simulink model "OMAP"  (R2018b)
settings: Solver=FixedStepDiscrete  StartTime=0.0  StopTime=10.0  FixedStep=0.01  RelTol=1e-3
values from neighbouring files (symbols this model uses):
  Clb_ICADirect_LaneDisp_StateFive = Simulink.Parameter    [omap_ver_442.m]
  Clb_ICADirect_LaneDisp_StateFour = Simulink.Parameter    [omap_ver_442.m]
  Clb_ICADirect_LaneDisp_StateOne = Simulink.Parameter    [omap_ver_442.m]
  Clb_ICADirect_LaneDisp_StateThree = Simulink.Parameter    [omap_ver_442.m]
  Clb_ICADirect_LaneDisp_StateTwo = Simulink.Parameter    [omap_ver_442.m]
  Clb_ICADirect_LaneDisp_StateZero = Simulink.Parameter    [omap_ver_442.m]
  Clb_ICADirect_LaneDispSW = Simulink.Parameter    [omap_ver_442.m]
  Clb_ICADirect_TrnLghtsCom_Switch = Simulink.Parameter    [omap_ver_442.m]
  Clb_ICADirect_TrnLghtsCom_Value = Simulink.Parameter    [omap_ver_442.m]
  Clb_ICADirect_TrnLghtsCrtl_Inhb = Simulink.Parameter    [omap_ver_442.m]
  OMAP_ACCAEB_EMSESC_Decel = Simulink.Parameter    [omap_ver_442.m]
  OMAP_ACCFCW_IC_Decel = Simulink.Parameter    [omap_ver_442.m]
  OMAP_clb_ACC_RVVReqType = Simulink.Parameter    [omap_ver_442.m]
  OMAP_clb_ACC_RVVReqType_Switch = Simulink.Parameter    [omap_ver_442.m]
  OMAP_clb_ACCHeadwayDisplay = Simulink.Parameter    [omap_ver_442.m]
  OMAP_clb_ACCHeadwayDisplay_Switch = Simulink.Parameter    [omap_ver_442.m]
  OMAP_clb_ACCHeadwayIcon = Simulink.Parameter    [omap_ver_442.m]
  OMAP_clb_ACCHeadwayIcon_Switch = Simulink.Parameter    [omap_ver_442.m]
  OMAP_clb_ACCMessagePrompt = Simulink.Parameter    [omap_ver_442.m]
  OMAP_clb_ACCMessagePrompt_Switch = Simulink.Parameter    [omap_ver_442.m]
  OMAP_clb_ACCRequestEPB = Simulink.Parameter    [omap_ver_442.m]
  OMAP_clb_ACCRequestEPB_Switch = Simulink.Parameter    [omap_ver_442.m]
  OMAP_clb_ACCSetSpeed = Simulink.Parameter    [omap_ver_442.m]
  OMAP_clb_ACCSetSpeed_Switch = Simulink.Parameter    [omap_ver_442.m]
  OMAP_clb_ACCSetSpeedDis = Simulink.Parameter    [omap_ver_442.m]
  OMAP_clb_ACCSetSpeedDis_Switch = Simulink.Parameter    [omap_ver_442.m]
  OMAP_clb_ACCState = Simulink.Parameter    [omap_ver_442.m]
  OMAP_clb_ACCState_Switch = Simulink.Parameter    [omap_ver_442.m]
  OMAP_clb_ACCStatusIconDis = Simulink.Parameter    [omap_ver_442.m]
  OMAP_clb_ACCStatusIconDis_Switch = Simulink.Parameter    [omap_ver_442.m]
  OMAP_clb_ACCTorqueReq = Simulink.Parameter    [omap_ver_442.m]
  OMAP_clb_ACCTorqueReq_Switch = Simulink.Parameter    [omap_ver_442.m]
  OMAP_clb_ADAS_State = Simulink.Parameter    [omap_ver_442.m]
  OMAP_clb_ADAS_State_Switch = Simulink.Parameter    [omap_ver_442.m]
  OMAP_clb_AEBAlertReq = Simulink.Parameter    [omap_ver_442.m]
  OMAP_clb_AEBAlertReq_Switch = Simulink.Parameter    [omap_ver_442.m]
  OMAP_clb_AEBBrakingProg = Simulink.Parameter    [omap_ver_442.m]
  OMAP_clb_AEBBrakingProg_Switch = Simulink.Parameter    [omap_ver_442.m]
  OMAP_clb_AEBFaultStatus = Simulink.Parameter    [omap_ver_442.m]
  OMAP_clb_AEBFaultStatus_Switch = Simulink.Parameter    [omap_ver_442.m]
  OMAP_clb_AEBMassageDisp = Simulink.Parameter    [omap_ver_442.m]
  OMAP_clb_AEBMassageDisp_Switch = Simulink.Parameter    [omap_ver_442.m]
  OMAP_clb_AEBState = Simulink.Parameter    [omap_ver_442.m]
  OMAP_clb_AEBState_Switch = Simulink.Parameter    [omap_ver_442.m]
  OMAP_clb_AEBSwitchStatus = Simulink.Parameter    [omap_ver_442.m]
  OMAP_clb_AEBSwitchStatus_Switch = Simulink.Parameter    [omap_ver_442.m]
  OMAP_clb_BrakeRequest = Simulink.Parameter    [omap_ver_442.m]
  OMAP_clb_BrakeRequest_Switch = Simulink.Parameter    [omap_ver_442.m]
  OMAP_clb_DecelerationSet = Simulink.Parameter    [omap_ver_442.m]
  OMAP_clb_DecelerationSet_Switch = Simulink.Parameter    [omap_ver_442.m]
  OMAP_clb_DecelerationType = Simulink.Parameter    [omap_ver_442.m]
  OMAP_clb_DecelerationType_Switch = Simulink.Parameter    [omap_ver_442.m]
  OMAP_clb_DeclControlReq = Simulink.Parameter    [omap_ver_442.m]
  OMAP_clb_DeclControlReq_Switch = Simulink.Parameter    [omap_ver_442.m]
  OMAP_clb_DownorUpGearMinTime = Simulink.Parameter    [omap_ver_442.m]
  OMAP_clb_DownorUpGearMinTime_Switch = Simulink.Parameter    [omap_ver_442.m]
  OMAP_clb_ELKPopupMessage = Simulink.Parameter    [omap_ver_442.m]
  OMAP_clb_ELKPopupMessage_Switch = Simulink.Parameter    [omap_ver_442.m]
  OMAP_clb_ELKSts = Simulink.Parameter    [omap_ver_442.m]
  OMAP_clb_ELKSts_Switch = Simulink.Parameter    [omap_ver_442.m]
  OMAP_clb_ESAFaultSt = Simulink.Parameter    [omap_ver_442.m]
  OMAP_clb_ESAFaultSt_Switch = Simulink.Parameter    [omap_ver_442.m]
  OMAP_clb_ESARequest = Simulink.Parameter    [omap_ver_442.m]
  OMAP_clb_ESARequest_Switch = Simulink.Parameter    [omap_ver_442.m]
  OMAP_clb_ESAState = Simulink.Parameter    [omap_ver_442.m]
  OMAP_clb_ESAState_Switch = Simulink.Parameter    [omap_ver_442.m]
  OMAP_clb_ESATorqueReq = Simulink.Parameter    [omap_ver_442.m]
  OMAP_clb_ESATorqueReq_Switch = Simulink.Parameter    [omap_ver_442.m]
  OMAP_clb_ESCDriveOff = Simulink.Parameter    [omap_ver_442.m]
  OMAP_clb_ESCDriveOff_Switch = Simulink.Parameter    [omap_ver_442.m]
  OMAP_clb_ESCHoldReq = Simulink.Parameter    [omap_ver_442.m]
  OMAP_clb_ESCHoldReq_Switch = Simulink.Parameter    [omap_ver_442.m]
  OMAP_clb_Handsoffwarning = Simulink.Parameter    [omap_ver_442.m]
  OMAP_clb_Handsoffwarning_Switch = Simulink.Parameter    [omap_ver_442.m]
  OMAP_clb_HapticAlarmReq = Simulink.Parameter    [omap_ver_442.m]
  OMAP_clb_HapticAlarmReq_Switch = Simulink.Parameter    [omap_ver_442.m]
  OMAP_clb_HMIPopupMassage = Simulink.Parameter    [omap_ver_442.m]
  OMAP_clb_HMIPopupMassage_Switch = Simulink.Parameter    [omap_ver_442.m]
  OMAP_clb_HWAActionSts = Simulink.Parameter    [omap_ver_442.m]
  OMAP_clb_HWAActionSts_Switch = Simulink.Parameter    [omap_ver_442.m]
  OMAP_clb_HWAMode = Simulink.Parameter    [omap_ver_442.m]
  OMAP_clb_HWAMode_Switch = Simulink.Parameter    [omap_ver_442.m]
  OMAP_clb_HWATurnOnIdctr = Simulink.Parameter    [omap_ver_442.m]
  OMAP_clb_HWATurnOnIdctr_Switch = Simulink.Parameter    [omap_ver_442.m]
  OMAP_clb_ICAMassageDisp = Simulink.Parameter    [omap_ver_442.m]
  OMAP_clb_ICAMassageDisp_Switch = Simulink.Parameter    [omap_ver_442.m]
  OMAP_clb_ICAStatusIcon = Simulink.Parameter    [omap_ver_442.m]
  OMAP_clb_ICAStatusIcon_Switch = Simulink.Parameter    [omap_ver_442.m]
  OMAP_clb_ISLCDriverRemind = Simulink.Parameter    [omap_ver_442.m]
  OMAP_clb_ISLCDriverRemind_Switch = Simulink.Parameter    [omap_ver_442.m]
  OMAP_clb_ISLCState = Simulink.Parameter    [omap_ver_442.m]
  OMAP_clb_ISLCState_Switch = Simulink.Parameter    [omap_ver_442.m]
  OMAP_clb_JAFaultSt = Simulink.Parameter    [omap_ver_442.m]
  OMAP_clb_JAFaultSt_Switch = Simulink.Parameter    [omap_ver_442.m]
  OMAP_clb_LCAPopupMessage = Simulink.Parameter    [omap_ver_442.m]
  OMAP_clb_LCAPopupMessage_Switch = Simulink.Parameter    [omap_ver_442.m]
  OMAP_clb_LCAStatusDisplay = Simulink.Parameter    [omap_ver_442.m]
  OMAP_clb_LCAStatusDisplay_Switch = Simulink.Parameter    [omap_ver_442.m]
  OMAP_clb_LDWStatusDisplay = Simulink.Parameter    [omap_ver_442.m]
  OMAP_clb_LDWStatusDisplay_Switch = Simulink.Parameter    [omap_ver_442.m]
  OMAP_clb_LDWWarningSt = Simulink.Parameter    [omap_ver_442.m]
  OMAP_clb_LDWWarningSt_Switch = Simulink.Parameter    [omap_ver_442.m]
  OMAP_clb_LightControlValid = Simulink.Parameter    [omap_ver_442.m]
  OMAP_clb_LightControlValid_Switch = Simulink.Parameter    [omap_ver_442.m]
  OMAP_clb_LKAActivation = Simulink.Parameter    [omap_ver_442.m]
  OMAP_clb_LKAActivation_Switch = Simulink.Parameter    [omap_ver_442.m]
  OMAP_clb_LKAAngleReq = Simulink.Parameter    [omap_ver_442.m]
  OMAP_clb_LKAAngleReq_Switch = Simulink.Parameter    [omap_ver_442.m]
  OMAP_clb_LKAMode = Simulink.Parameter    [omap_ver_442.m]
  OMAP_clb_LKAMode_Switch = Simulink.Parameter    [omap_ver_442.m]
  OMAP_clb_LKAorELK_CoolTime = Simulink.Parameter    [omap_ver_442.m]
  OMAP_clb_LKAState = Simulink.Parameter    [omap_ver_442.m]
  OMAP_clb_LKAState_Switch = Simulink.Parameter    [omap_ver_442.m]
  OMAP_clb_LKAStatusDisplay = Simulink.Parameter    [omap_ver_442.m]
  OMAP_clb_LKAStatusDisplay_Switch = Simulink.Parameter    [omap_ver_442.m]
  OMAP_clb_LKASwitchState = Simulink.Parameter    [omap_ver_442.m]
  OMAP_clb_LKASwitchState_Switch = Simulink.Parameter    [omap_ver_442.m]
  OMAP_clb_LKATorqFactReq = Simulink.Parameter    [omap_ver_442.m]
  OMAP_clb_LKATorqFactReq_Switch = Simulink.Parameter    [omap_ver_442.m]
  OMAP_clb_PrefillRequest = Simulink.Parameter    [omap_ver_442.m]
  ... (+36 more)
libraries: simulink x184, canmsglib x2
(part 14 of 14)

== system OMAP/Runnable_OMAP_10ms_sys/OMAP_Module/ICA_Direct_G59/ICA_Define/Subsystem1/Dspl/DsplPrcs/Txt/TxtFromACC/RdrBlkInhib ==
  RdrBlkInhib_stTHState : Inport
  RdrBlkInhib_stLstTHState : Inport  Port=2
  RdrBlkInhib_stACCTxtDspl : Inport  Port=3
  Constant1 : Constant  OutDataTypeStr=uint16
  Constant2 : Constant  Value=0  OutDataTypeStr=uint16
  If : If  NumInputs=3  IfExpression=u1 == 5 & u2 == 0 & u3 == 2  ElseIfExpressions=u1 ~= 5 | u3 ~= 2
  Inhibit : Subsystem  TreatAsAtomicUnit=on
  Merge : Merge  Inputs=3
  Unit Delay1 : UnitDelay  SampleTime=-1
  hold_last : Subsystem  TreatAsAtomicUnit=on
  not_Inhibit : Subsystem  TreatAsAtomicUnit=on
  RdrBlkInhib_stRdrBlkInhibFlg : Outport
  wires:
  RdrBlkInhib_stTHState/1 -> If/1
  Merge/1 -> Unit Delay1/1, RdrBlkInhib_stRdrBlkInhibFlg/1
  Inhibit/1(Out1) -> Merge/1
  RdrBlkInhib_stLstTHState/1 -> If/2
  RdrBlkInhib_stACCTxtDspl/1 -> If/3
  Constant1/1 -> Inhibit/1(In1)
  If/1 -> Inhibit/Action
  Constant2/1 -> not_Inhibit/1(In1)
  If/2 -> not_Inhibit/Action
  Unit Delay1/1 -> hold_last/1(In1)
  If/3 -> hold_last/Action
  not_Inhibit/1(Out1) -> Merge/2
  hold_last/1(Out1) -> Merge/3

== system OMAP/Runnable_OMAP_10ms_sys/OMAP_Module/ICA_Direct_G59/ICA_Define/Subsystem1/Dspl/DsplPrcs/Txt/TxtFromACC/Start ==
  In1 : Inport
  Action Port : ActionPort  ActionType=then
  Out1 : Outport
  wires:
  In1/1 -> Out1/1

== system OMAP/Runnable_OMAP_10ms_sys/OMAP_Module/ICA_Direct_G59/ICA_Define/Subsystem1/Dspl/DsplPrcs/Txt/TxtFromACC/Start1 ==
  In1 : Inport
  Action Port : ActionPort  ActionType=then
  Out1 : Outport
  wires:
  In1/1 -> Out1/1

== system OMAP/Runnable_OMAP_10ms_sys/OMAP_Module/ICA_Direct_G59/ICA_Define/Subsystem1/Dspl/DsplPrcs/Txt/TxtFromACC/Start2 ==
  In1 : Inport
  Action Port : ActionPort  ActionType=then
  Out1 : Outport
  wires:
  In1/1 -> Out1/1

== system OMAP/Runnable_OMAP_10ms_sys/OMAP_Module/ICA_Direct_G59/ICA_Define/Subsystem1/Dspl/DsplPrcs/Txt/TxtFromACC/Start3 ==
  In1 : Inport
  Action Port : ActionPort  ActionType=then
  Out1 : Outport
  wires:
  In1/1 -> Out1/1

== system OMAP/Runnable_OMAP_10ms_sys/OMAP_Module/ICA_Direct_G59/ICA_Define/Subsystem1/Dspl/DsplPrcs/Txt/TxtFromACC/Start4 ==
  In1 : Inport
  Action Port : ActionPort  ActionType=then
  Out1 : Outport
  wires:
  In1/1 -> Out1/1

== system OMAP/Runnable_OMAP_10ms_sys/OMAP_Module/ICA_Direct_G59/ICA_Define/Subsystem1/Dspl/DsplPrcs/Txt/TxtFromACC/Start5 ==
  In1 : Inport
  Action Port : ActionPort  ActionType=then
  Out1 : Outport
  wires:
  In1/1 -> Out1/1

== system OMAP/Runnable_OMAP_10ms_sys/OMAP_Module/ICA_Direct_G59/ICA_Define/Subsystem1/Dspl/DsplPrcs/Txt/TxtFromACC/Start6 ==
  In1 : Inport
  Action Port : ActionPort  ActionType=then
  Out1 : Outport
  wires:
  In1/1 -> Out1/1

== system OMAP/Runnable_OMAP_10ms_sys/OMAP_Module/ICA_Direct_G59/ICA_Define/Subsystem1/Dspl/DsplPrcs/Txt/TxtFromACC/Start7 ==
  In1 : Inport
  Action Port : ActionPort  ActionType=then
  Out1 : Outport
  wires:
  In1/1 -> Out1/1

== system OMAP/Runnable_OMAP_10ms_sys/OMAP_Module/ICA_Direct_G59/ICA_Define/Subsystem1/Dspl/DsplPrcs/Txt/TxtFromACC/Start8 ==
  In1 : Inport
  Action Port : ActionPort  ActionType=then
  Out1 : Outport
  wires:
  In1/1 -> Out1/1

== system OMAP/Runnable_OMAP_10ms_sys/OMAP_Module/ICA_Direct_G59/ICA_Define/Subsystem1/Dspl/DsplPrcs/Txt/TxtFromACC/Start9 ==
  In1 : Inport
  Action Port : ActionPort  ActionType=then
  Out1 : Outport
  wires:
  In1/1 -> Out1/1

== system OMAP/Runnable_OMAP_10ms_sys/OMAP_Module/ICA_Direct_G59/ICA_Define/Subsystem1/Dspl/DsplPrcs/Txt/TxtFromACC/Stop ==
  In1 : Inport
  Action Port : ActionPort  ActionType=else
  Out1 : Outport
  wires:
  In1/1 -> Out1/1

== system OMAP/Runnable_OMAP_10ms_sys/OMAP_Module/ICA_Direct_G59/ICA_Define/Subsystem1/Dspl/DsplPrcs/Txt/TxtFromACC/Stop1 ==
  In1 : Inport
  Action Port : ActionPort  ActionType=else
  Out1 : Outport
  wires:
  In1/1 -> Out1/1

== system OMAP/Runnable_OMAP_10ms_sys/OMAP_Module/ICA_Direct_G59/ICA_Define/Subsystem1/Dspl/DsplPrcs/Txt/TxtFromACC/Stop2 ==
  In1 : Inport
  Action Port : ActionPort  ActionType=else
  Out1 : Outport
  wires:
  In1/1 -> Out1/1

== system OMAP/Runnable_OMAP_10ms_sys/OMAP_Module/ICA_Direct_G59/ICA_Define/Subsystem1/Dspl/DsplPrcs/Txt/TxtFromACC/Stop3 ==
  In1 : Inport
  Action Port : ActionPort  ActionType=else
  Out1 : Outport
  wires:
  In1/1 -> Out1/1

== system OMAP/Runnable_OMAP_10ms_sys/OMAP_Module/ICA_Direct_G59/ICA_Define/Subsystem1/Dspl/DsplPrcs/Txt/TxtFromACC/Stop4 ==
  In1 : Inport
  Action Port : ActionPort  ActionType=elseif
  Out1 : Outport
  wires:
  In1/1 -> Out1/1

== system OMAP/Runnable_OMAP_10ms_sys/OMAP_Module/ICA_Direct_G59/ICA_Define/Subsystem1/Dspl/DsplPrcs/Txt/TxtFromACC/Stop5 ==
  In1 : Inport
  Action Port : ActionPort  ActionType=else
  Out1 : Outport
  wires:
  In1/1 -> Out1/1

== system OMAP/Runnable_OMAP_10ms_sys/OMAP_Module/ICA_Direct_G59/ICA_Define/Subsystem1/Dspl/DsplPrcs/Txt/TxtFromACC/Stop6 ==
  In1 : Inport
  Action Port : ActionPort  ActionType=else
  Out1 : Outport
  wires:
  In1/1 -> Out1/1

== system OMAP/Runnable_OMAP_10ms_sys/OMAP_Module/ICA_Direct_G59/ICA_Define/Subsystem1/Dspl/DsplPrcs/Txt/TxtFromACC/Stop7 ==
  In1 : Inport
  Action Port : ActionPort  ActionType=else
  Out1 : Outport
  wires:
  In1/1 -> Out1/1

== system OMAP/Runnable_OMAP_10ms_sys/OMAP_Module/ICA_Direct_G59/ICA_Define/Subsystem1/Dspl/DsplPrcs/Txt/TxtFromACC/Stop8 ==
  In1 : Inport
  Action Port : ActionPort  ActionType=else
  Out1 : Outport
  wires:
  In1/1 -> Out1/1

== system OMAP/Runnable_OMAP_10ms_sys/OMAP_Module/ICA_Direct_G59/ICA_Define/Subsystem1/Dspl/DsplPrcs/Txt/TxtFromACC/Stop9 ==
  In1 : Inport
  Action Port : ActionPort  ActionType=else
  Out1 : Outport
  wires:
  In1/1 -> Out1/1

== system OMAP/Runnable_OMAP_10ms_sys/OMAP_Module/ICA_Direct_G59/ICA_Define/Subsystem1/Dspl/DsplPrcs/Txt/TxtInactv/Hold ==
  In1 : Inport
  Action Port : ActionPort  ActionType=else
  Out1 : Outport
  wires:
  In1/1 -> Out1/1

== system OMAP/Runnable_OMAP_10ms_sys/OMAP_Module/ICA_Direct_G59/ICA_Define/Subsystem1/Dspl/DsplPrcs/Txt/TxtInactv/Start ==
  In1 : Inport
  Action Port : ActionPort  ActionType=elseif
  Out1 : Outport
  wires:
  In1/1 -> Out1/1

== system OMAP/Runnable_OMAP_10ms_sys/OMAP_Module/ICA_Direct_G59/ICA_Define/Subsystem1/Dspl/DsplPrcs/Txt/TxtInactv/Stop ==
  In1 : Inport
  Action Port : ActionPort  ActionType=then
  Out1 : Outport
  wires:
  In1/1 -> Out1/1

== system OMAP/Runnable_OMAP_10ms_sys/OMAP_Module/ICA_Direct_G59/ICA_Define/Subsystem1/Dspl/DsplPrcs/Txt/TxtOff/Hold ==
  In1 : Inport
  Action Port : ActionPort  ActionType=else
  Out1 : Outport
  wires:
  In1/1 -> Out1/1

== system OMAP/Runnable_OMAP_10ms_sys/OMAP_Module/ICA_Direct_G59/ICA_Define/Subsystem1/Dspl/DsplPrcs/Txt/TxtOff/Start ==
  In1 : Inport
  Action Port : ActionPort  ActionType=then
  Out1 : Outport
  wires:
  In1/1 -> Out1/1

== system OMAP/Runnable_OMAP_10ms_sys/OMAP_Module/ICA_Direct_G59/ICA_Define/Subsystem1/Dspl/DsplPrcs/Txt/TxtOff/Stop ==
  In1 : Inport
  Action Port : ActionPort  ActionType=elseif
  Out1 : Outport
  wires:
  In1/1 -> Out1/1

== system OMAP/Runnable_OMAP_10ms_sys/OMAP_Module/ICA_Direct_G59/ICA_Define/Subsystem1/Dspl/DsplPrcs/Txt/TxtOffToFault/Hold ==
  In1 : Inport
  Action Port : ActionPort  ActionType=else
  Out1 : Outport
  wires:
  In1/1 -> Out1/1

== system OMAP/Runnable_OMAP_10ms_sys/OMAP_Module/ICA_Direct_G59/ICA_Define/Subsystem1/Dspl/DsplPrcs/Txt/TxtOffToFault/Start ==
  In1 : Inport
  Action Port : ActionPort  ActionType=then
  Out1 : Outport
  wires:
  In1/1 -> Out1/1

== system OMAP/Runnable_OMAP_10ms_sys/OMAP_Module/ICA_Direct_G59/ICA_Define/Subsystem1/Dspl/DsplPrcs/Txt/TxtOffToFault/Stop ==
  In1 : Inport
  Action Port : ActionPort  ActionType=elseif
  Out1 : Outport
  wires:
  In1/1 -> Out1/1

== system OMAP/Runnable_OMAP_10ms_sys/OMAP_Module/ICA_Direct_G59/ICA_Define/Subsystem1/Dspl/DsplPrcs/Txt/TxtOn/Hold ==
  In1 : Inport
  Action Port : ActionPort  ActionType=else
  Out1 : Outport
  wires:
  In1/1 -> Out1/1

== system OMAP/Runnable_OMAP_10ms_sys/OMAP_Module/ICA_Direct_G59/ICA_Define/Subsystem1/Dspl/DsplPrcs/Txt/TxtOn/Start ==
  In1 : Inport
  Action Port : ActionPort  ActionType=then
  Out1 : Outport
  wires:
  In1/1 -> Out1/1

== system OMAP/Runnable_OMAP_10ms_sys/OMAP_Module/ICA_Direct_G59/ICA_Define/Subsystem1/Dspl/DsplPrcs/Txt/TxtOn/Stop ==
  In1 : Inport
  Action Port : ActionPort  ActionType=elseif
  Out1 : Outport
  wires:
  In1/1 -> Out1/1

== system OMAP/Runnable_OMAP_10ms_sys/OMAP_Module/ICA_Direct_G59/ICA_Define/Subsystem1/Dspl/DsplPrcs/Txt/TxtOnToFault/Hold ==
  In1 : Inport
  Action Port : ActionPort  ActionType=else
  Out1 : Outport
  wires:
  In1/1 -> Out1/1

== system OMAP/Runnable_OMAP_10ms_sys/OMAP_Module/ICA_Direct_G59/ICA_Define/Subsystem1/Dspl/DsplPrcs/Txt/TxtOnToFault/Start ==
  In1 : Inport
  Action Port : ActionPort  ActionType=then
  Out1 : Outport
  wires:
  In1/1 -> Out1/1

== system OMAP/Runnable_OMAP_10ms_sys/OMAP_Module/ICA_Direct_G59/ICA_Define/Subsystem1/Dspl/DsplPrcs/Txt/TxtOnToFault/Stop ==
  In1 : Inport
  Action Port : ActionPort  ActionType=elseif
  Out1 : Outport
  wires:
  In1/1 -> Out1/1

== system OMAP/Runnable_OMAP_10ms_sys/OMAP_Module/ICA_Direct_G59/ICA_Define/Subsystem1/Dspl/DsplPrcs/Txt/Txt_Tlimit/Hold ==
  In1 : Inport
  Action Port : ActionPort  ActionType=else
  Out1 : Outport
  wires:
  In1/1 -> Out1/1

== system OMAP/Runnable_OMAP_10ms_sys/OMAP_Module/ICA_Direct_G59/ICA_Define/Subsystem1/Dspl/DsplPrcs/Txt/Txt_Tlimit/Start ==
  In1 : Inport
  Action Port : ActionPort  ActionType=then
  Out1 : Outport
  wires:
  In1/1 -> Out1/1

== system OMAP/Runnable_OMAP_10ms_sys/OMAP_Module/ICA_Direct_G59/ICA_Define/Subsystem1/Dspl/DsplPrcs/Txt/Txt_Tlimit/Stop ==
  In1 : Inport
  Action Port : ActionPort  ActionType=elseif
  Out1 : Outport
  wires:
  In1/1 -> Out1/1

== system OMAP/Runnable_OMAP_10ms_sys/OMAP_Module/ICA_Direct_G59/ICA_Define/Subsystem1/Dspl/DsplPrcs/Txt/Txt_Tlimit1/Hold ==
  In1 : Inport
  Action Port : ActionPort  ActionType=else
  Out1 : Outport
  wires:
  In1/1 -> Out1/1

== system OMAP/Runnable_OMAP_10ms_sys/OMAP_Module/ICA_Direct_G59/ICA_Define/Subsystem1/Dspl/DsplPrcs/Txt/Txt_Tlimit1/Start ==
  In1 : Inport
  Action Port : ActionPort  ActionType=then
  Out1 : Outport
  wires:
  In1/1 -> Out1/1

== system OMAP/Runnable_OMAP_10ms_sys/OMAP_Module/ICA_Direct_G59/ICA_Define/Subsystem1/Dspl/DsplPrcs/Txt/Txt_Tlimit1/Stop ==
  In1 : Inport
  Action Port : ActionPort  ActionType=elseif
  Out1 : Outport
  wires:
  In1/1 -> Out1/1

== system OMAP/Runnable_OMAP_10ms_sys/OMAP_Module/ICA_Direct_G59/ICA_Define/Subsystem1/Dspl/DsplPrcs/Txt/Txt_Tlimit2/Hold ==
  In1 : Inport
  Action Port : ActionPort  ActionType=else
  Out1 : Outport
  wires:
  In1/1 -> Out1/1

== system OMAP/Runnable_OMAP_10ms_sys/OMAP_Module/ICA_Direct_G59/ICA_Define/Subsystem1/Dspl/DsplPrcs/Txt/Txt_Tlimit2/Start ==
  In1 : Inport
  Action Port : ActionPort  ActionType=then
  Out1 : Outport
  wires:
  In1/1 -> Out1/1

== system OMAP/Runnable_OMAP_10ms_sys/OMAP_Module/ICA_Direct_G59/ICA_Define/Subsystem1/Dspl/DsplPrcs/Txt/Txt_Tlimit2/Stop ==
  In1 : Inport
  Action Port : ActionPort  ActionType=elseif
  Out1 : Outport
  wires:
  In1/1 -> Out1/1

== system OMAP/Runnable_OMAP_10ms_sys/OMAP_Module/ICA_Direct_G59/ICA_Define/Subsystem1/Dspl/DsplPrcs/Txt/Txt_Tlimit3/Hold ==
  In1 : Inport
  Action Port : ActionPort  ActionType=else
  Out1 : Outport
  wires:
  In1/1 -> Out1/1

== system OMAP/Runnable_OMAP_10ms_sys/OMAP_Module/ICA_Direct_G59/ICA_Define/Subsystem1/Dspl/DsplPrcs/Txt/Txt_Tlimit3/Start ==
  In1 : Inport
  Action Port : ActionPort  ActionType=then
  Out1 : Outport
  wires:
  In1/1 -> Out1/1

== system OMAP/Runnable_OMAP_10ms_sys/OMAP_Module/ICA_Direct_G59/ICA_Define/Subsystem1/Dspl/DsplPrcs/Txt/Txt_Tlimit3/Stop ==
  In1 : Inport
  Action Port : ActionPort  ActionType=elseif
  Out1 : Outport
  wires:
  In1/1 -> Out1/1

== system OMAP/Runnable_OMAP_10ms_sys/OMAP_Module/ICA_Direct_G59/ICA_Define/Subsystem1/Dspl/DsplPrcs/Txt/Txt_Tlimit4/Hold ==
  In1 : Inport
  Action Port : ActionPort  ActionType=else
  Out1 : Outport
  wires:
  In1/1 -> Out1/1

== system OMAP/Runnable_OMAP_10ms_sys/OMAP_Module/ICA_Direct_G59/ICA_Define/Subsystem1/Dspl/DsplPrcs/Txt/Txt_Tlimit4/Start ==
  In1 : Inport
  Action Port : ActionPort  ActionType=then
  Out1 : Outport
  wires:
  In1/1 -> Out1/1

== system OMAP/Runnable_OMAP_10ms_sys/OMAP_Module/ICA_Direct_G59/ICA_Define/Subsystem1/Dspl/DsplPrcs/Txt/Txt_Tlimit4/Stop ==
  In1 : Inport
  Action Port : ActionPort  ActionType=elseif
  Out1 : Outport
  wires:
  In1/1 -> Out1/1

== system OMAP/Runnable_OMAP_10ms_sys/OMAP_Module/ICA_Direct_G59/ICA_Define/Subsystem1/Dspl/DsplPrcs/Txt/Txt_Tlimit5/Hold ==
  In1 : Inport
  Action Port : ActionPort  ActionType=else
  Out1 : Outport
  wires:
  In1/1 -> Out1/1

== system OMAP/Runnable_OMAP_10ms_sys/OMAP_Module/ICA_Direct_G59/ICA_Define/Subsystem1/Dspl/DsplPrcs/Txt/Txt_Tlimit5/Start ==
  In1 : Inport
  Action Port : ActionPort  ActionType=then
  Out1 : Outport
  wires:
  In1/1 -> Out1/1

== system OMAP/Runnable_OMAP_10ms_sys/OMAP_Module/ICA_Direct_G59/ICA_Define/Subsystem1/Dspl/DsplPrcs/Txt/Txt_Tlimit5/Stop ==
  In1 : Inport
  Action Port : ActionPort  ActionType=elseif
  Out1 : Outport
  wires:
  In1/1 -> Out1/1

== system OMAP/Runnable_OMAP_10ms_sys/OMAP_Module/ICA_Direct_G59/ICA_Define/Subsystem1/Dspl/DsplPrcs/Txt/Txt_Tlimit6/Hold ==
  In1 : Inport
  Action Port : ActionPort  ActionType=else
  Out1 : Outport
  wires:
  In1/1 -> Out1/1

== system OMAP/Runnable_OMAP_10ms_sys/OMAP_Module/ICA_Direct_G59/ICA_Define/Subsystem1/Dspl/DsplPrcs/Txt/Txt_Tlimit6/Start ==
  In1 : Inport
  Action Port : ActionPort  ActionType=then
  Out1 : Outport
  wires:
  In1/1 -> Out1/1

== system OMAP/Runnable_OMAP_10ms_sys/OMAP_Module/ICA_Direct_G59/ICA_Define/Subsystem1/Dspl/DsplPrcs/Txt/Txt_Tlimit6/Stop ==
  In1 : Inport
  Action Port : ActionPort  ActionType=elseif
  Out1 : Outport
  wires:
  In1/1 -> Out1/1

== system OMAP/Runnable_OMAP_10ms_sys/OMAP_Module/ICA_Direct_G59/ICA_Define/Subsystem1/Dspl/DsplPrcs/Txt/Txt_Tlimit7/Hold ==
  In1 : Inport
  Action Port : ActionPort  ActionType=else
  Out1 : Outport
  wires:
  In1/1 -> Out1/1

== system OMAP/Runnable_OMAP_10ms_sys/OMAP_Module/ICA_Direct_G59/ICA_Define/Subsystem1/Dspl/DsplPrcs/Txt/Txt_Tlimit7/Start ==
  In1 : Inport
  Action Port : ActionPort  ActionType=then
  Out1 : Outport
  wires:
  In1/1 -> Out1/1

== system OMAP/Runnable_OMAP_10ms_sys/OMAP_Module/ICA_Direct_G59/ICA_Define/Subsystem1/Dspl/DsplPrcs/Txt/Txt_Tlimit7/Stop ==
  In1 : Inport
  Action Port : ActionPort  ActionType=elseif
  Out1 : Outport
  wires:
  In1/1 -> Out1/1

== system OMAP/Runnable_OMAP_10ms_sys/OMAP_Module/ICA_Direct_G59/ICA_Define/Subsystem1/Dspl/DsplPrcs/Txt/TxtFromACC/RdrBlkInhib/Inhibit ==
  In1 : Inport
  Action Port : ActionPort  ActionType=then
  Out1 : Outport
  wires:
  In1/1 -> Out1/1

== system OMAP/Runnable_OMAP_10ms_sys/OMAP_Module/ICA_Direct_G59/ICA_Define/Subsystem1/Dspl/DsplPrcs/Txt/TxtFromACC/RdrBlkInhib/hold_last ==
  In1 : Inport
  Action Port : ActionPort  ActionType=else
  Out1 : Outport
  wires:
  In1/1 -> Out1/1

== system OMAP/Runnable_OMAP_10ms_sys/OMAP_Module/ICA_Direct_G59/ICA_Define/Subsystem1/Dspl/DsplPrcs/Txt/TxtFromACC/RdrBlkInhib/not_Inhibit ==
  In1 : Inport
  Action Port : ActionPort  ActionType=elseif
  Out1 : Outport
  wires:
  In1/1 -> Out1/1

== stateflow chart OMAP/Runnable_OMAP_10ms_sys/OMAP_Module/ACCS_Direct/ACCS_Define/ACC_State_Synthesis(ACC_SS)/If Action Subsystem2/Subsystem4/Chart ==
  state Zero
    en:
    RAPPORT=uint8(0);
  state One
    en:
    RAPPORT=uint8(1);
  (default) -> Zero
  Zero -> One : [after(2,tick)]
  One -> Zero : [[after(2,tick)]]
  data: RAPPORT output uint8

== stateflow chart OMAP/Runnable_OMAP_10ms_sys/OMAP_Module/ACCS_Direct/ACCS_Define/ACC_State_Synthesis(ACC_SS)/If Action Subsystem3/Subsystem6/Chart ==
  state Zero
    en:
    RAPPORT=uint8(0);
  state One
    en:
    RAPPORT=uint8(1);
  (default) -> Zero
  Zero -> One : [after(2,tick)]
  One -> Zero : [after(2,tick)]
  data: RAPPORT output uint8

== stateflow chart OMAP/Runnable_OMAP_10ms_sys/OMAP_Module/Subsystem/IC_Arbitration/LKA_arb_ELK/Subsystem/Chart1 ==
  state ELK_Action
    en:
    state = uint8(2);
  state Default
    en:
    state = uint8(1);
  state LKA_Action
    en:
    state = uint8(1);
  state LKA_cooling
    en:
    state = uint8(1);
  state ELK_cooling
    en:
    state = uint8(2);
  (default) -> (junction 1)
  (junction 1) -> ELK_Action [order 1] : [ELK_Up&&(~LKA_Up)]
  (junction 48) -> (junction 1) : [~LKA_Active&&~ELK_Active]
  (junction 1) -> Default [order 2]
  Default -> ELK_Action [order 2] : [ELK_Up]
  (junction 41) -> ELK_Action [order 1] : [ELK_Up]
  ELK_Action -> ELK_cooling : [ELK_Down]
  Default -> LKA_Action [order 1] : [LKA_Up]
  (junction 30) -> LKA_Action [order 2] : [LKA_Up]
  LKA_Action -> LKA_cooling : [LKA_Down]
  LKA_cooling -> (junction 30)
  ELK_cooling -> (junction 41)
  (junction 30) -> (junction 48) [order 1] : [after(cool_time,sec)]
  (junction 41) -> (junction 48) [order 2] : [after(cool_time,sec)]
  data: LKA_Up input boolean; LKA_Down input boolean; LKA_Active input boolean; ELK_Up input boolean; ELK_Down input boolean; ELK_Active input boolean; state output uint8; cool_time input single

== matlab function OMAP/Runnable_OMAP_10ms_sys/OMAP_Module/Subsystem/IC_Arbitration/ACC_ICA/MATLAB Function ==
  data: ACC_Message input; ACC_Message_out output; ICA_Message input; ICA_Message_out output
function [ACC_Message_out,ICA_Message_out] = fcn(ACC_Message, ICA_Message)
if ACC_Message == uint16(1) && ICA_Message == uint8(11)
    ACC_Message_out = uint16(1);
    ICA_Message_out = uint8(0);
elseif ACC_Message == uint16(10) && ICA_Message == uint8(1)
    ACC_Message_out = uint16(0);
    ICA_Message_out = uint8(1);
else
    ACC_Message_out = ACC_Message;
    ICA_Message_out = ICA_Message;
end

== stateflow chart OMAP/Runnable_OMAP_10ms_sys/OMAP_Module/Subsystem/EPS_Default_Arbitration/LKA_arb_ELK/Subsystem2/Chart1 ==
  state ELK_Action
    en:
    state = uint8(2);
  state Default
    en:
    state = uint8(1);
  state LKA_Action
    en:
    state = uint8(1);
  state LKA_cooling
    en:
    state = uint8(1);
  state ELK_cooling
    en:
    state = uint8(2);
  (default) -> (junction 1)
  (junction 1) -> ELK_Action [order 1] : [ELK_Up&&(~LKA_Up)]
  (junction 48) -> (junction 1) : [~LKA_Active&&~ELK_Active]
  (junction 1) -> Default [order 2]
  Default -> ELK_Action [order 2] : [ELK_Up]
  (junction 41) -> ELK_Action [order 1] : [ELK_Up]
  ELK_Action -> ELK_cooling : [ELK_Down]
  Default -> LKA_Action [order 1] : [LKA_Up]
  (junction 30) -> LKA_Action [order 2] : [LKA_Up]
  LKA_Action -> LKA_cooling : [LKA_Down]
  LKA_cooling -> (junction 30)
  ELK_cooling -> (junction 41)
  (junction 30) -> (junction 48) [order 1] : [after(cool_time,sec)]
  (junction 41) -> (junction 48) [order 2] : [after(cool_time,sec)]
  data: LKA_Up input boolean; LKA_Down input boolean; LKA_Active input boolean; ELK_Up input boolean; ELK_Down input boolean; ELK_Active input boolean; state output uint8; cool_time input single

== matlab function OMAP/Runnable_OMAP_10ms_sys/OMAP_Module/ICA_Direct_G59/ICA_Define/ICA_EPS/EPS_Ctr_Disable/MATLAB Function ==
  data: stEPSCtlState input; stEPSCtlCMD output; ControlCMDdisable input
function stEPSCtlCMD = fcn(stEPSCtlState, ControlCMDdisable)
    stEPSCtlCMD=ControlCMDdisable;  %select
end

== matlab function OMAP/Runnable_OMAP_10ms_sys/OMAP_Module/ICA_Direct_G59/ICA_Define/ICA_EPS/EPS_Ctr_Enable/MATLAB Function ==
  data: stEPSCtlState input; stEPSCtlCMD output; EPSCMDselect input; EPSCMDauthorized input; EPSCMDactive input
function stEPSCtlCMD = fcn(stEPSCtlState, EPSCMDselect, EPSCMDauthorized, EPSCMDactive)
if stEPSCtlState==uint16(0) %unauthorized
    stEPSCtlCMD=EPSCMDselect;  %select
elseif stEPSCtlState==uint16(2) %available
    stEPSCtlCMD=EPSCMDauthorized;  %authorized
elseif stEPSCtlState==uint16(1) %authorized
    stEPSCtlCMD=EPSCMDactive;  %active
elseif stEPSCtlState==uint16(3) %active
    stEPSCtlCMD=EPSCMDactive;  %active
else
    stEPSCtlCMD=EPSCMDselect;  %select
end

== matlab function OMAP/Runnable_OMAP_10ms_sys/OMAP_Module/ACCS_Direct/ACCS_Define/CIPV_Data ==
  data: IMAPva_d_obj_id input; IMAPva_g_obj_pos_x input; ACCSve_d_CIPV_ID input; CIPV_ID_Longitudinal_Distance output
function CIPV_ID_Longitudinal_Distance = CIPV_Data(IMAPva_d_obj_id, IMAPva_g_obj_pos_x, ACCSve_d_CIPV_ID)
%%依据CIPV_ID求出对应的纵向距离
%分类有目标和无目标
%依据CIPV_ID值求解其在IMAPva_d_obj_id的index
CIPV_ID_Longitudinal_Distance = single(200);

if ACCSve_d_CIPV_ID ~= 0
    for i = 1:40
        if IMAPva_d_obj_id(i) == ACCSve_d_CIPV_ID
            CIPV_ID_Longitudinal_Distance = IMAPva_g_obj_pos_x(i);
        end
    end
end
end

== matlab function OMAP/Runnable_OMAP_10ms_sys/OMAP_Module/ICA_Direct_G59/ICA_Define/Subsystem1/Count1 ==
  data: count_out output
function count_out = fcn()
%#codegen
persistent count;
if isempty(count)
    count=uint16(0);
end
count=count+uint16(1);
if count>=uint16(300)
    count=uint16(0);
end
count_out = count;

== matlab function OMAP/Runnable_OMAP_10ms_sys/OMAP_Module/ICA_Direct_G59/ICA_Define/Subsystem1/Dspl/DsplPrcs/Txt/PrioPrcs ==
  data: HndOffFlg input; GoReqFlg input; THState input; PrioPrcs_TxtDspl output; OffFlg input; TkOvFlg input; ImmdTkOvFlg input; RdrBlkFlg input; OnToFaultFlg input; OffToFaultFlg input; CnclFlg input; OnFlg input; ActvFlg input; InactvFlg input; DegradedFlg input; PressSetFlg input; ResEPBFlg input; ResBrkPedalFlg input; ISAToOnFlg input; ISAToOffFlg input
function PrioPrcs_TxtDspl  = fcn(HndOffFlg,GoReqFlg, THState,OffFlg,TkOvFlg,ImmdTkOvFlg,RdrBlkFlg,OnToFaultFlg,OffToFaultFlg,CnclFlg,OnFlg,ActvFlg,InactvFlg,DegradedFlg,PressSetFlg, ResEPBFlg, ResBrkPedalFlg, ISAToOnFlg, ISAToOffFlg)
if(ImmdTkOvFlg == uint16(1))
    PrioPrcs_TxtDspl = uint16(9);%% Please take over the car immediately %%
elseif ((THState ~= uint16(0))&&(THState ~= uint16(5))&&(HndOffFlg == 1))
    PrioPrcs_TxtDspl = uint16(8);%% Please hold the steering wheel %%
elseif (TkOvFlg == uint16(1))
    PrioPrcs_TxtDspl = uint16(7);%% Please take over the car %%
elseif (GoReqFlg == uint16(1))
    PrioPrcs_TxtDspl = uint16(6);%% ICA go request %%
elseif (OnToFaultFlg == uint16(1))
    PrioPrcs_TxtDspl = uint16(3);%% ICA Fault %%
elseif (OffToFaultFlg == uint16(1))
    PrioPrcs_TxtDspl = uint16(3);%% ICA Fault %%
elseif (RdrBlkFlg == uint16(1))
    PrioPrcs_TxtDspl = uint16(2);%% Radar Blocked %%
elseif (OffFlg == uint16(1))
    PrioPrcs_TxtDspl = uint16(11);%% ICA OFF %%
elseif (CnclFlg == uint16(1))
    PrioPrcs_TxtDspl = uint16(10);%% ICA Canceled %%    
elseif (ActvFlg == uint16(1))
    PrioPrcs_TxtDspl = uint16(5);%% ICA Active %%
elseif (ResBrkPedalFlg == uint16(1))
    PrioPrcs_TxtDspl = uint16(15);%% Release BRAKE PEDAL then active Intelligent Cruise Assist  %%
elseif (ResEPBFlg == uint16(1))
    PrioPrcs_TxtDspl = uint16(14);%% Release EPB then reactive Intelligent Cruise Assist   %%
elseif (PressSetFlg == uint16(1))
    PrioPrcs_TxtDspl = uint16(13);%% SET- key to active Intelligent Cruise Assist    %%
elseif (InactvFlg == uint16(1))
    PrioPrcs_TxtDspl = uint16(4);%% Intelligent Cruise Assist System Activation Unsatisfied %%
elseif (OnFlg == uint16(1))
    PrioPrcs_TxtDspl = uint16(1);%% Intelligent Cruise Assist System ON %%
elseif (ISAToOnFlg == uint16(1))
    PrioPrcs_TxtDspl = uint16(16);%% Temporary speed down %%
elseif (ISAToOffFlg == uint16(1))
    PrioPrcs_TxtDspl = uint16(17);%% Accelerating to target speed %%
elseif (DegradedFlg == uint16(1))
    PrioPrcs_TxtDspl = uint16(12);%% ICA degraded %%
else
    PrioPrcs_TxtDspl = uint16(0);%% No_display %%
end

== matlab function OMAP/Runnable_OMAP_10ms_sys/OMAP_Module/ICA_Direct_G59/ICA_Define/Subsystem1/Dspl/DsplPrcs/Voc/MATLAB_Function ==
  data: Warning_duration input; Warning output; Trigger input
function Warning = fcn(Warning_duration,Trigger)
%#codegen
persistent count;
if isempty(count)
    count=uint16(0);
end
if Trigger==uint16(1)
    count=Warning_duration;
end
if count>=uint16(1)
    count=count-uint16(1);
end
if count==uint16(0)
    Warning=uint16(0);
else
    Warning=uint16(1);
end
end

== matlab function OMAP/Runnable_OMAP_10ms_sys/OMAP_Module/ICA_Direct_G59/ICA_Define/Subsystem1/Subsystem/MATLAB Function ==
  data: TH_Mode input; LC_Scene input; TSR_Version_Only_Sign_Type output; stLCRMode input
function TSR_Version_Only_Sign_Type = fcn(TH_Mode,LC_Scene,stLCRMode)
Left_Turn=uint16(16);
Right_Turn=uint16(15);
No_Turn=uint16(0);
ZERO=uint16(0);
ONE=uint16(1);
TWO=uint16(2);
THREE=uint16(3);
if(TH_Mode~=uint16(4))
    if(stLCRMode==TWO)
        TSR_Version_Only_Sign_Type=Left_Turn;
    elseif(stLCRMode==THREE)
        TSR_Version_Only_Sign_Type=Right_Turn;   
    else
        TSR_Version_Only_Sign_Type=No_Turn;   
    end
else
    if(LC_Scene==ONE)  %Left
       TSR_Version_Only_Sign_Type=Left_Turn;
    elseif(LC_Scene==TWO)
        TSR_Version_Only_Sign_Type=Right_Turn;   
    else
        TSR_Version_Only_Sign_Type=No_Turn;  
    end
end
end

== stateflow chart OMAP/Runnable_OMAP_10ms_sys/OMAP_Module/ACCS_Direct/ACCS_Define/Human_Machine_Interface(ACC_HMI)/Subsystem/Chart ==
  state ObjOutRange
    en:
    Value = uint8(5);
  state ObjInRange
    state Middle
      en:
      Value = uint8(2);
    state Far
      en:
      Value = uint8(4);
    state Close
      en:
      Value = uint8(1);
    (default) -> (junction 14)
    (junction 14) -> Far [order 2] : [Distance>single(80)]
    (junction 14) -> Close [order 1] : [Distance<=single(30)]
    (junction 14) -> Middle [order 3]
    Far -> Middle [order 1] : [(Distance>single(30))&&(Distance<single(77))]
    Middle -> Close [order 1] : [Distance<single(27)]
    Middle -> Far [order 2] : [Distance>single(80)]
    Close -> Middle [order 1] : [(Distance>single(30))&&(Distance<=single(80))]
    Close -> Far [order 2] : [Distance>single(80)]
    Far -> Close [order 2] : [Distance<=single(30)]
  (default) -> (junction 28)
  (junction 28) -> ObjInRange [order 1] : [(Distance>=single(0))&&(Distance<=single(150))]
  (junction 28) -> ObjOutRange [order 2]
  ObjInRange -> ObjOutRange : [(Distance<single(0))||(Distance>single(150))]
  ObjOutRange -> ObjInRange : [(Distance>=single(0))&&(Distance<=single(150))]
  data: Distance input; Value output uint8

== stateflow chart OMAP/Runnable_OMAP_10ms_sys/OMAP_Module/ACCS_Direct/ACCS_Define/Human_Machine_Interface(ACC_HMI)/Text_PopUp/ Radar_Blocked/Chart ==
  state StandBy
    en:
    Value = data;
  state Trigger
    en:
    Value = data;
  (default) -> StandBy
  StandBy -> Trigger : [data==1]
  Trigger -> StandBy : [after(3,sec)]
  data: data input; Value output boolean

== stateflow chart OMAP/Runnable_OMAP_10ms_sys/OMAP_Module/ACCS_Direct/ACCS_Define/Human_Machine_Interface(ACC_HMI)/Text_PopUp/ACC_Activation_Unsatisfied/Chart ==
  state StandBy
    en:
    Value = data;
  state Trigger
    en:
    Value = data;
  (default) -> StandBy
  StandBy -> Trigger : [data==1]
  Trigger -> StandBy : [after(3,sec)]
  data: data input; Value output boolean

== stateflow chart OMAP/Runnable_OMAP_10ms_sys/OMAP_Module/ACCS_Direct/ACCS_Define/Human_Machine_Interface(ACC_HMI)/Text_PopUp/ACC_Active/Chart ==
  state StandBy
    en:
    Value = data;
  state Trigger
    en:
    Value = data;
  (default) -> StandBy
  StandBy -> Trigger : [data==1]
  Trigger -> StandBy : [after(3,sec)]
  data: data input; Value output boolean

== stateflow chart OMAP/Runnable_OMAP_10ms_sys/OMAP_Module/ACCS_Direct/ACCS_Define/Human_Machine_Interface(ACC_HMI)/Text_PopUp/ACC_Canceled/Chart ==
  state StandBy
    en:
    Value = data;
  state Trigger
    en:
    Value = data;
  (default) -> StandBy
  StandBy -> Trigger : [data==1]
  Trigger -> StandBy : [after(3,sec)]
  data: data input; Value output boolean

== stateflow chart OMAP/Runnable_OMAP_10ms_sys/OMAP_Module/ACCS_Direct/ACCS_Define/Human_Machine_Interface(ACC_HMI)/Text_PopUp/ACC_Fault/Chart ==
  state StandBy
    en:
    Value = data;
  state Trigger
    en:
    Value = data;
  (default) -> StandBy
  StandBy -> Trigger : [data==1]
  Trigger -> StandBy : [after(3,sec)]
  data: data input; Value output boolean

== stateflow chart OMAP/Runnable_OMAP_10ms_sys/OMAP_Module/ACCS_Direct/ACCS_Define/Human_Machine_Interface(ACC_HMI)/Text_PopUp/ACC_OFF/Chart ==
  state StandBy
    en:
    Value = data;
  state Trigger
    en:
    Value = data;
  (default) -> StandBy
  StandBy -> Trigger : [(data==1)&&(data1==0)]
  Trigger -> StandBy : [after(3,sec)]
  data: data input; Value output boolean; data1 input

== stateflow chart OMAP/Runnable_OMAP_10ms_sys/OMAP_Module/ACCS_Direct/ACCS_Define/Human_Machine_Interface(ACC_HMI)/Text_PopUp/ACC_ON/Chart ==
  state StandBy
    en:
    Value = data;
  state Trigger
    en:
    Value = data;
  state Trigger1
    en:
    Value = data2;
  (default) -> StandBy
  StandBy -> Trigger [order 1] : [data==1]
  Trigger -> StandBy : [after(6,sec)||(data1==1)]
  Trigger1 -> StandBy : [after(6,sec)||(data1==1)]
  StandBy -> Trigger1 [order 2] : [data2==1]
  data: data input; Value output boolean; data1 input; data2 input

== stateflow chart OMAP/Runnable_OMAP_10ms_sys/OMAP_Module/ACCS_Direct/ACCS_Define/Human_Machine_Interface(ACC_HMI)/Text_PopUp/Please_Take_Over_the_Car/Chart1 ==
  state StandBy
    en:
    Value = uint8(0);
  state Trigger
    en:
    Value = uint8(1);
  (default) -> StandBy
  StandBy -> Trigger : [IN==1]
  Trigger -> StandBy : [OUT==1]
  data: IN input boolean; OUT input boolean; Value output uint8

== stateflow chart OMAP/Runnable_OMAP_10ms_sys/OMAP_Module/ACCS_Direct/ACCS_Define/Human_Machine_Interface(ACC_HMI)/Text_PopUp/Please_Take_Over_the_Car_immediataly/Chart1 ==
  state StandBy1
    en:
    Value = uint8(0);
  state Trigger
    en:
    Value = uint8(1);
  state StandBy
    en:
    Value = uint8(0);
  (default) -> StandBy
  StandBy -> StandBy1 : [(ESC_DecTar>-5)&&(ESC_DecTar<-3)]
  StandBy1 -> Trigger [order 2] : [after(4,sec)]
  StandBy1 -> StandBy [order 1] : [ESC_DecTar>-3]
  Trigger -> StandBy : [ESC_DecTar>-3]
  data: ESC_DecTar input single; Value output uint8; BRAKE_RELEASED_FAILSAFE input
